simulink model "SimscapeCrane_MPChard"  (R2015b)
settings: Solver=ode15s  StartTime=0.0  StopTime=T  RelTol=1e-3
values from neighbouring files (symbols this model uses):
  m = m1/N    [ConstraintMatrices.m]
  N = N1/(n+c)    [SoftPadding.m]    (also in testMPC.m = ceil(Tf/Ts); testMyLP.m = ceil(1.5/Ts); testRHC.m = ceil(1.5/Ts))
  s = size(A)    [Prediction.m]
  Ts = 1.5/10    (= 0.15)    [testMPC.m]    (also in testMyLP.m; testRHC.m)
  xTarget = [xRange(2)*0.8 0 xRange(2)*0.8 0 0 0 0 0]'    [testMyLP.m]
  xZero = xRange(2)*0.05    [testMPC.m]    (also in testRHC.m = 0)
  yZero = yRange(2)*0.05    [testMPC.m]    (also in testRHC.m = 0)
undefined symbols (not defined in the file or in its folder): Al, blx0, blxe, CD, Dx0, MR, TxBreak, TxCoulomb, TxVisc, TyBreak, TyCoulomb, TzBreak, TzCoulomb, ucon, X, xRange, Y, yRange, Z, zRange, zZero
undefined symbols (not defined in the file): M, TorqueMultX, TorqueMultY, TorqueMultZ, TxTrans, TyTrans, TyVisc, TzTrans, TzVisc
libraries: sm_lib x146, fl_lib x62, nesl_utility x24, elec_lib x9, simulink x6, sm_double_wishbone_suspension_lib x4, aerolibtransform2 x1
(part 14 of 14)

== system SimscapeCrane_MPChard/Crane1/XY actuator/DC Y/PWM & H-Bridge1/Vr Scope ==
  Electrical Reference1 : fl_lib/Electrical/Electrical Elements/Electrical Reference
  PS-Simulink Converter 2 : nesl_utility/PS-Simulink Converter  PhysicalDomain=network_engine_domain  SubClassName=ps_output  LeftPortType=input  RightPortType=output  PseudoPeriodic=off  Frequencies=[]  Unit=V  AffineConversion=off
  Voltage Sensor : fl_lib/Electrical/Electrical Sensors/Voltage Sensor
  Vr : Scope
  u : PMIOPort  Port=1  Side=Left
  wires:
  PS-Simulink Converter 2/1 -> Vr/1
  connections:
  u/RConn1 -- Voltage Sensor/LConn1
  Voltage Sensor/RConn1 -- PS-Simulink Converter 2/LConn1
  Voltage Sensor/RConn2 -- Electrical Reference1/LConn1

== system SimscapeCrane_MPChard/Crane1/XY actuator/X rail/DC X/PWM & H-Bridge ==
  note: For validation purposes the simulation mode
      | can be set to PWM in both the Controlled PWM
      | and H-Bridge blocks.
  Controlled PWM Voltage : elec_lib/Actuators & Drivers/Drivers/Controlled PWM Voltage  F=10000 Hz  TD=0 s  pulse_width_offset=0 s  Vmin=0 V  Vmax=5 V  Vm=5 V  pwm_or_av=2  event_type=1  sample_time=1e-6 s
  Electrical Reference2 : fl_lib/Electrical/Electrical Elements/Electrical Reference
  H-Bridge : elec_lib/Actuators & Drivers/Drivers/H-Bridge  Venable=2.5 V  Vmax=5 V  Vreverse=2.5 V  Vbrake=2.5 V  Vm=24 V  pwm_or_av=2  discontinuous=0  freewheeling_mode=1  freewheeling_mode_disc=1  Ron=0.1 Ohm  Don=0.1 Ohm  Rload=10 Ohm  Lload=1e-5 H  F=10 kHz  thermal_mass=100 J/K  initial_temperature=298.15 K  Ron2=0.1 Ohm  Don2=0.05 Ohm  Tmeas=298.15 K  Tmeas2=398.15 K
  PWM Scope : Subsystem
  REV Scope : Subsystem  Commented=on
  Vr Scope : Subsystem  Commented=on
  V+ : PMIOPort  Port=1  Side=Right
  V- : PMIOPort  Port=2  Side=Right
  Vr : PMIOPort  Port=3  Side=Left
  REV : PMIOPort  Port=4  Side=Left
  "brk " : PMIOPort  Port=5  Side=Left
  "gnd " : PMIOPort  Port=6  Side=Left
  connections:
  V+/RConn1 -- H-Bridge/RConn1
  H-Bridge/RConn2 -- V-/RConn1 -- Electrical Reference2/LConn1
  PWM Scope/LConn1 -- H-Bridge/LConn1 -- Controlled PWM Voltage/RConn1
  Vr Scope/LConn1 -- Controlled PWM Voltage/LConn1 -- Vr/RConn1
  REV Scope/LConn1 -- H-Bridge/LConn3 -- REV/RConn1
  H-Bridge/LConn2 -- Controlled PWM Voltage/RConn2 -- Controlled PWM Voltage/LConn2 -- "gnd "/RConn1
  "brk "/RConn1 -- H-Bridge/LConn4

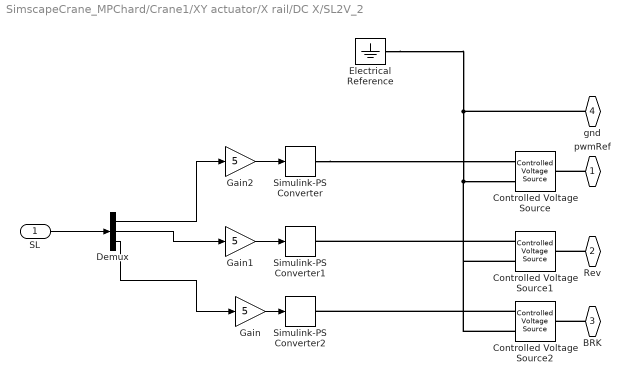
== system SimscapeCrane_MPChard/Crane1/XY actuator/X rail/DC X/SL2V_2 ==
  SL : Inport
  Controlled Voltage Source : fl_lib/Electrical/Electrical Sources/Controlled Voltage Source
  Controlled Voltage Source1 : fl_lib/Electrical/Electrical Sources/Controlled Voltage Source
  Controlled Voltage Source2 : fl_lib/Electrical/Electrical Sources/Controlled Voltage Source
  Demux : Demux  Outputs=3
  Electrical Reference : fl_lib/Electrical/Electrical Elements/Electrical Reference
  Gain : Gain  Gain=5
  Gain1 : Gain  Gain=5
  Gain2 : Gain  Gain=5
  Simulink-PS Converter : nesl_utility/Simulink-PS Converter  PhysicalDomain=network_engine_domain  SubClassName=ps_input  LeftPortType=input  RightPortType=output  PseudoPeriodic=off  Frequencies=[]  NoiseDistribution=none  NoiseParameters=[]  Unit=V  AffineConversion=off  InputFiltering=off  SimscapeFilterOrder=1  InputFilterTimeConstant=.001  UdotUserProvided=0
  Simulink-PS Converter1 : nesl_utility/Simulink-PS Converter  PhysicalDomain=network_engine_domain  SubClassName=ps_input  LeftPortType=input  RightPortType=output  PseudoPeriodic=off  Frequencies=[]  NoiseDistribution=none  NoiseParameters=[]  Unit=V  AffineConversion=off  InputFiltering=off  SimscapeFilterOrder=1  InputFilterTimeConstant=.001  UdotUserProvided=0
  Simulink-PS Converter2 : nesl_utility/Simulink-PS Converter  PhysicalDomain=network_engine_domain  SubClassName=ps_input  LeftPortType=input  RightPortType=output  PseudoPeriodic=off  Frequencies=[]  NoiseDistribution=none  NoiseParameters=[]  Unit=V  AffineConversion=off  InputFiltering=off  SimscapeFilterOrder=1  InputFilterTimeConstant=.001  UdotUserProvided=0
  pwmRef : PMIOPort  Port=1  Side=Right
  Rev : PMIOPort  Port=2  Side=Right
  BRK : PMIOPort  Port=3  Side=Right
  "gnd " : PMIOPort  Port=4  Side=Right
  wires:
  SL/1 -> Demux/1
  Demux/1 -> Gain2/1
  Demux/3 -> Gain/1
  Gain/1 -> Simulink-PS Converter2/1
  Demux/2 -> Gain1/1
  Gain1/1 -> Simulink-PS Converter1/1
  Gain2/1 -> Simulink-PS Converter/1
  connections:
  Simulink-PS Converter/RConn1 -- Controlled Voltage Source/RConn1
  pwmRef/RConn1 -- Controlled Voltage Source/LConn1
  Electrical Reference/LConn1 -- "gnd "/RConn1 -- Controlled Voltage Source/RConn2 -- Controlled Voltage Source1/RConn2 -- Controlled Voltage Source2/RConn2
  Rev/RConn1 -- Controlled Voltage Source1/LConn1
  Controlled Voltage Source2/RConn1 -- Simulink-PS Converter2/RConn1
  BRK/RConn1 -- Controlled Voltage Source2/LConn1
  Controlled Voltage Source1/RConn1 -- Simulink-PS Converter1/RConn1

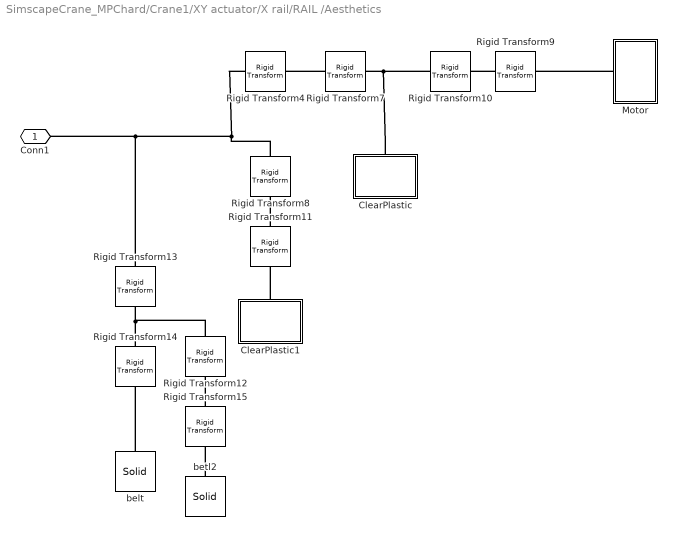
== system SimscapeCrane_MPChard/Crane1/XY actuator/X rail/RAIL /Aesthetics ==
  ClearPlastic : Subsystem
  ClearPlastic1 : Subsystem
  Motor : Subsystem
  Rigid Transform10 : sm_lib/Frames and Transforms/Rigid Transform  TranslationMethod=StandardAxis  TranslationLengthUnit=m  TranslationStandardAxis=+X  TranslationStandardOffset=0.03  TranslationCartesianOffset="[-0.5 0  0]"  TranslationROffset=0  TranslationROffsetUnits=m  TranslationZOffset=0  TranslationZOffsetUnits=m  TranslationThetaOffset=0  TranslationThetaOffsetUnits=deg  RotationMethod=None  RotationAngleUnits=deg  RotationStandardAxis=+Y  RotationAngle=90  RotationArbitraryAxis=[0 0 1]  FollAlignAxisA=+X  BaseAlignAxisA=+Y  FollAlignAxisB=+Y  BaseAlignAxisB=+Z  RotationSequenceAxes=FollowerAxes  RotationSequence=XYX  RotationSequenceAngles=[0 0 0]  RotationSequenceAnglesUnits=deg  RotationMatrix=[1 0 0; 0 1 0; 0 0 1]  BlockFunction=simmechanics.library.frames_transforms.rigid_transform
  Rigid Transform11 : sm_lib/Frames and Transforms/Rigid Transform  TranslationMethod=StandardAxis  TranslationLengthUnit=m  TranslationStandardAxis=-Z  TranslationStandardOffset=0.05  TranslationCartesianOffset="[-0.5 0  0]"  TranslationROffset=0  TranslationROffsetUnits=m  TranslationZOffset=0  TranslationZOffsetUnits=m  TranslationThetaOffset=0  TranslationThetaOffsetUnits=deg  RotationMethod=None  RotationAngleUnits=deg  RotationStandardAxis=+Y  RotationAngle=90  RotationArbitraryAxis=[0 0 1]  FollAlignAxisA=+X  BaseAlignAxisA=+Y  FollAlignAxisB=+Y  BaseAlignAxisB=+Z  RotationSequenceAxes=FollowerAxes  RotationSequence=XYX  RotationSequenceAngles=[0 0 0]  RotationSequenceAnglesUnits=deg  RotationMatrix=[1 0 0; 0 1 0; 0 0 1]  BlockFunction=simmechanics.library.frames_transforms.rigid_transform
  Rigid Transform12 : sm_lib/Frames and Transforms/Rigid Transform  TranslationMethod=StandardAxis  TranslationLengthUnit=m  TranslationStandardAxis=-Z  TranslationStandardOffset=0.06  TranslationCartesianOffset="[-0.5 0  0]"  TranslationROffset=0  TranslationROffsetUnits=m  TranslationZOffset=0  TranslationZOffsetUnits=m  TranslationThetaOffset=0  TranslationThetaOffsetUnits=deg  RotationMethod=None  RotationAngleUnits=deg  RotationStandardAxis=+Y  RotationAngle=90  RotationArbitraryAxis=[0 0 1]  FollAlignAxisA=+X  BaseAlignAxisA=+Y  FollAlignAxisB=+Y  BaseAlignAxisB=+Z  RotationSequenceAxes=FollowerAxes  RotationSequence=XYX  RotationSequenceAngles=[0 0 0]  RotationSequenceAnglesUnits=deg  RotationMatrix=[1 0 0; 0 1 0; 0 0 1]  BlockFunction=simmechanics.library.frames_transforms.rigid_transform
  Rigid Transform13 : sm_lib/Frames and Transforms/Rigid Transform  TranslationMethod=StandardAxis  TranslationLengthUnit=m  TranslationStandardAxis=-X  TranslationStandardOffset=0.04  TranslationCartesianOffset="[-0.5 0  0]"  TranslationROffset=0  TranslationROffsetUnits=m  TranslationZOffset=0  TranslationZOffsetUnits=m  TranslationThetaOffset=0  TranslationThetaOffsetUnits=deg  RotationMethod=None  RotationAngleUnits=deg  RotationStandardAxis=+Y  RotationAngle=90  RotationArbitraryAxis=[0 0 1]  FollAlignAxisA=+X  BaseAlignAxisA=+Y  FollAlignAxisB=+Y  BaseAlignAxisB=+Z  RotationSequenceAxes=FollowerAxes  RotationSequence=XYX  RotationSequenceAngles=[0 0 0]  RotationSequenceAnglesUnits=deg  RotationMatrix=[1 0 0; 0 1 0; 0 0 1]  BlockFunction=simmechanics.library.frames_transforms.rigid_transform
  Rigid Transform14 : sm_lib/Frames and Transforms/Rigid Transform  TranslationMethod=None  TranslationLengthUnit=m  TranslationStandardAxis=-Z  TranslationStandardOffset=0.04  TranslationCartesianOffset="[-0.5 0  0]"  TranslationROffset=0  TranslationROffsetUnits=m  TranslationZOffset=0  TranslationZOffsetUnits=m  TranslationThetaOffset=0  TranslationThetaOffsetUnits=deg  RotationMethod=StandardAxis  RotationAngleUnits=deg  RotationStandardAxis=+Z  RotationAngle=90  RotationArbitraryAxis=[0 0 1]  FollAlignAxisA=+X  BaseAlignAxisA=+Y  FollAlignAxisB=+Y  BaseAlignAxisB=+Z  RotationSequenceAxes=FollowerAxes  RotationSequence=XYX  RotationSequenceAngles=[0 0 0]  RotationSequenceAnglesUnits=deg  RotationMatrix=[1 0 0; 0 1 0; 0 0 1]  BlockFunction=simmechanics.library.frames_transforms.rigid_transform
  Rigid Transform15 : sm_lib/Frames and Transforms/Rigid Transform  TranslationMethod=None  TranslationLengthUnit=m  TranslationStandardAxis=-Z  TranslationStandardOffset=0.04  TranslationCartesianOffset="[-0.5 0  0]"  TranslationROffset=0  TranslationROffsetUnits=m  TranslationZOffset=0  TranslationZOffsetUnits=m  TranslationThetaOffset=0  TranslationThetaOffsetUnits=deg  RotationMethod=StandardAxis  RotationAngleUnits=deg  RotationStandardAxis=+Z  RotationAngle=90  RotationArbitraryAxis=[0 0 1]  FollAlignAxisA=+X  BaseAlignAxisA=+Y  FollAlignAxisB=+Y  BaseAlignAxisB=+Z  RotationSequenceAxes=FollowerAxes  RotationSequence=XYX  RotationSequenceAngles=[0 0 0]  RotationSequenceAnglesUnits=deg  RotationMatrix=[1 0 0; 0 1 0; 0 0 1]  BlockFunction=simmechanics.library.frames_transforms.rigid_transform
  Rigid Transform4 : sm_lib/Frames and Transforms/Rigid Transform  TranslationMethod=StandardAxis  TranslationLengthUnit=m  TranslationStandardAxis=-Y  TranslationStandardOffset=0.56  TranslationCartesianOffset="[-0.5 0  0]"  TranslationROffset=0  TranslationROffsetUnits=m  TranslationZOffset=0  TranslationZOffsetUnits=m  TranslationThetaOffset=0  TranslationThetaOffsetUnits=deg  RotationMethod=None  RotationAngleUnits=deg  RotationStandardAxis=+Y  RotationAngle=90  RotationArbitraryAxis=[0 0 1]  FollAlignAxisA=+X  BaseAlignAxisA=+Y  FollAlignAxisB=+Y  BaseAlignAxisB=+Z  RotationSequenceAxes=FollowerAxes  RotationSequence=XYX  RotationSequenceAngles=[0 0 0]  RotationSequenceAnglesUnits=deg  RotationMatrix=[1 0 0; 0 1 0; 0 0 1]  BlockFunction=simmechanics.library.frames_transforms.rigid_transform
  Rigid Transform7 : sm_lib/Frames and Transforms/Rigid Transform  TranslationMethod=StandardAxis  TranslationLengthUnit=m  TranslationStandardAxis=-Z  TranslationStandardOffset=0.05  TranslationCartesianOffset="[-0.5 0  0]"  TranslationROffset=0  TranslationROffsetUnits=m  TranslationZOffset=0  TranslationZOffsetUnits=m  TranslationThetaOffset=0  TranslationThetaOffsetUnits=deg  RotationMethod=None  RotationAngleUnits=deg  RotationStandardAxis=+Y  RotationAngle=90  RotationArbitraryAxis=[0 0 1]  FollAlignAxisA=+X  BaseAlignAxisA=+Y  FollAlignAxisB=+Y  BaseAlignAxisB=+Z  RotationSequenceAxes=FollowerAxes  RotationSequence=XYX  RotationSequenceAngles=[0 0 0]  RotationSequenceAnglesUnits=deg  RotationMatrix=[1 0 0; 0 1 0; 0 0 1]  BlockFunction=simmechanics.library.frames_transforms.rigid_transform
  Rigid Transform8 : sm_lib/Frames and Transforms/Rigid Transform  TranslationMethod=StandardAxis  TranslationLengthUnit=m  TranslationStandardAxis=+Y  TranslationStandardOffset=0.56  TranslationCartesianOffset="[-0.5 0  0]"  TranslationROffset=0  TranslationROffsetUnits=m  TranslationZOffset=0  TranslationZOffsetUnits=m  TranslationThetaOffset=0  TranslationThetaOffsetUnits=deg  RotationMethod=None  RotationAngleUnits=deg  RotationStandardAxis=+Y  RotationAngle=90  RotationArbitraryAxis=[0 0 1]  FollAlignAxisA=+X  BaseAlignAxisA=+Y  FollAlignAxisB=+Y  BaseAlignAxisB=+Z  RotationSequenceAxes=FollowerAxes  RotationSequence=XYX  RotationSequenceAngles=[0 0 0]  RotationSequenceAnglesUnits=deg  RotationMatrix=[1 0 0; 0 1 0; 0 0 1]  BlockFunction=simmechanics.library.frames_transforms.rigid_transform
  Rigid Transform9 : sm_lib/Frames and Transforms/Rigid Transform  TranslationMethod=None  TranslationLengthUnit=m  TranslationStandardAxis=-Z  TranslationStandardOffset=0.05  TranslationCartesianOffset="[-0.5 0  0]"  TranslationROffset=0  TranslationROffsetUnits=m  TranslationZOffset=0  TranslationZOffsetUnits=m  TranslationThetaOffset=0  TranslationThetaOffsetUnits=deg  RotationMethod=StandardAxis  RotationAngleUnits=deg  RotationStandardAxis=+Z  RotationAngle=90  RotationArbitraryAxis=[0 0 1]  FollAlignAxisA=+X  BaseAlignAxisA=+Y  FollAlignAxisB=+Y  BaseAlignAxisB=+Z  RotationSequenceAxes=FollowerAxes  RotationSequence=XYX  RotationSequenceAngles=[0 0 0]  RotationSequenceAnglesUnits=deg  RotationMatrix=[1 0 0; 0 1 0; 0 0 1]  BlockFunction=simmechanics.library.frames_transforms.rigid_transform
  belt : sm_lib/Body Elements/Solid  InertiaType=PointMass  Mass=0  MassUnits=kg  CenterOfMass=[0 0 0]  CenterOfMassUnits=m  MomentsOfInertia=[1 1 1]  MomentsOfInertiaUnits=kg*m^2  ProductsOfInertia=[0 0 0]  ProductsOfInertiaUnits=kg*m^2  DensityBased=off  Density=1000  DensityUnits=kg/(m^3)  DoExposeReferenceFrame=on  SerializedFrames=<Frames/>  GraphicType=FromGeometry  MarkerShape=Sphere  MarkerSize=10  MarkerSizeUnits=m  GraphicVisPropType=SimpleVisualProperties  GraphicDiffuseColor=[0.0 0.0 0.8]  GraphicSpecularColor=[0.5 0.5 0.5 1.0]  GraphicAmbientColor=[0.15 0.15 0.15 1.0]  GraphicEmissiveColor=[0.0 0.0 0.0 1.0]  GraphicShininess=100  GraphicOpacity=1.0  GeometryShape=Brick  RectangleSize=[1 1]  RectangleSizeUnits=m  BrickDimensions=[1.2 0.001 0.001]  BrickDimensionUnits=m  CylinderRadius=0.02  CylinderRadiusUnits=m  CylinderLength=1  CylinderLengthUnits=m  SphereRadius=1  SphereRadiusUnits=m  EllipsoidRadii=[1 1 1]  EllipsoidRadiiUnits=m  ExtrusionCrossSection=[1 1; -1 1; -1 -1; 1 -1]  ExtrusionCrossSectionUnits=m  ExtrusionLength=1  ExtrusionLengthUnits=m  PolygonNumSides=3  PolygonOuterRadius=1  PolygonOuterRadiusUnits=m  ExtGeomFileType=STL  ExtGeomFileUnits=m  RevolutionCrossSection=[1 1; 1 -1; 2 -1; 2 1]  RevolutionCrossSectionUnits=m  RevolutionExtent=Full  RevolutionAngle=180  RevolutionAngleUnits=deg  BlockFunction=simmechanics.library.body_elements.solid
  "betl2 " : sm_lib/Body Elements/Solid  InertiaType=PointMass  Mass=0  MassUnits=kg  CenterOfMass=[0 0 0]  CenterOfMassUnits=m  MomentsOfInertia=[1 1 1]  MomentsOfInertiaUnits=kg*m^2  ProductsOfInertia=[0 0 0]  ProductsOfInertiaUnits=kg*m^2  DensityBased=off  Density=1000  DensityUnits=kg/(m^3)  DoExposeReferenceFrame=on  SerializedFrames=<Frames/>  GraphicType=FromGeometry  MarkerShape=Sphere  MarkerSize=10  MarkerSizeUnits=m  GraphicVisPropType=SimpleVisualProperties  GraphicDiffuseColor=[0.0 0.0 0.8]  GraphicSpecularColor=[0.5 0.5 0.5 1.0]  GraphicAmbientColor=[0.15 0.15 0.15 1.0]  GraphicEmissiveColor=[0.0 0.0 0.0 1.0]  GraphicShininess=100  GraphicOpacity=1.0  GeometryShape=Brick  RectangleSize=[1 1]  RectangleSizeUnits=m  BrickDimensions=[1.2 0.001 0.001]  BrickDimensionUnits=m  CylinderRadius=0.02  CylinderRadiusUnits=m  CylinderLength=1  CylinderLengthUnits=m  SphereRadius=1  SphereRadiusUnits=m  EllipsoidRadii=[1 1 1]  EllipsoidRadiiUnits=m  ExtrusionCrossSection=[1 1; -1 1; -1 -1; 1 -1]  ExtrusionCrossSectionUnits=m  ExtrusionLength=1  ExtrusionLengthUnits=m  PolygonNumSides=3  PolygonOuterRadius=1  PolygonOuterRadiusUnits=m  ExtGeomFileType=STL  ExtGeomFileUnits=m  RevolutionCrossSection=[1 1; 1 -1; 2 -1; 2 1]  RevolutionCrossSectionUnits=m  RevolutionExtent=Full  RevolutionAngle=180  RevolutionAngleUnits=deg  BlockFunction=simmechanics.library.body_elements.solid
  Conn1 : PMIOPort  Port=1  Side=Left
  connections:
  Rigid Transform10/LConn1 -- ClearPlastic/RConn1 -- Rigid Transform7/RConn1
  Rigid Transform13/RConn1 -- Rigid Transform14/LConn1 -- Rigid Transform12/LConn1
  Motor/LConn1 -- Rigid Transform9/RConn1
  Rigid Transform7/LConn1 -- Rigid Transform4/RConn1
  ClearPlastic1/RConn1 -- Rigid Transform11/RConn1
  Rigid Transform11/LConn1 -- Rigid Transform8/RConn1
  Rigid Transform15/LConn1 -- Rigid Transform12/RConn1
  "betl2 "/RConn1 -- Rigid Transform15/RConn1
  Rigid Transform8/LConn1 -- Rigid Transform13/LConn1 -- Conn1/RConn1 -- Rigid Transform4/LConn1
  belt/RConn1 -- Rigid Transform14/RConn1
  Rigid Transform9/LConn1 -- Rigid Transform10/RConn1

== system SimscapeCrane_MPChard/Crane1/XY actuator/Y cart/CART/Motor ==
  Cart2 : sm_lib/Body Elements/Solid  InertiaType=PointMass  Mass=0  MassUnits=kg  CenterOfMass=[0 0 0]  CenterOfMassUnits=m  MomentsOfInertia=[1 1 1]  MomentsOfInertiaUnits=kg*m^2  ProductsOfInertia=[0 0 0]  ProductsOfInertiaUnits=kg*m^2  DensityBased=off  Density=1000  DensityUnits=kg/(m^3)  DoExposeReferenceFrame=on  SerializedFrames=<Frames/>  GraphicType=FromGeometry  MarkerShape=Sphere  MarkerSize=10  MarkerSizeUnits=m  GraphicVisPropType=AdvancedVisualProperties  GraphicDiffuseColor=[0.1 0.1 0.0]  GraphicSpecularColor=[0.5 0.5 0.5 1.0]  GraphicAmbientColor=[0.15 0.2 0.3 1.0]  GraphicEmissiveColor=[0.0 0.0 0.0 1.0]  GraphicShininess=30  GraphicOpacity=1.0  GeometryShape=Cylinder  RectangleSize=[1 1]  RectangleSizeUnits=m  BrickDimensions=[0.06 0.12 0.12]  BrickDimensionUnits=m  CylinderRadius=1.7  CylinderRadiusUnits=cm  CylinderLength=6  CylinderLengthUnits=cm  SphereRadius=1  SphereRadiusUnits=m  EllipsoidRadii=[1 1 1]  EllipsoidRadiiUnits=m  ExtrusionCrossSection=[1 1; -1 1; -1 -1; 1 -1]  ExtrusionCrossSectionUnits=m  ExtrusionLength=1  ExtrusionLengthUnits=m  PolygonNumSides=3  PolygonOuterRadius=1  PolygonOuterRadiusUnits=m  ExtGeomFileType=STL  ExtGeomFileUnits=m  RevolutionCrossSection=[1 1; 1 -1; 2 -1; 2 1]  RevolutionCrossSectionUnits=m  RevolutionExtent=Full  RevolutionAngle=180  RevolutionAngleUnits=deg  BlockFunction=simmechanics.library.body_elements.solid
  Cart3 : sm_lib/Body Elements/Solid  InertiaType=PointMass  Mass=0  MassUnits=kg  CenterOfMass=[0 0 0]  CenterOfMassUnits=m  MomentsOfInertia=[1 1 1]  MomentsOfInertiaUnits=kg*m^2  ProductsOfInertia=[0 0 0]  ProductsOfInertiaUnits=kg*m^2  DensityBased=off  Density=1000  DensityUnits=kg/(m^3)  DoExposeReferenceFrame=on  SerializedFrames=<Frames/>  GraphicType=FromGeometry  MarkerShape=Sphere  MarkerSize=10  MarkerSizeUnits=m  GraphicVisPropType=SimpleVisualProperties  GraphicDiffuseColor=[0.4 0.4 0.4]  GraphicSpecularColor=[0.5 0.5 0.5 1.0]  GraphicAmbientColor=[0.15 0.15 0.15 1.0]  GraphicEmissiveColor=[0.0 0.0 0.0 1.0]  GraphicShininess=75  GraphicOpacity=1.0  GeometryShape=Cylinder  RectangleSize=[1 1]  RectangleSizeUnits=m  BrickDimensions=[0.06 0.12 0.12]  BrickDimensionUnits=m  CylinderRadius=2.6  CylinderRadiusUnits=cm  CylinderLength=3  CylinderLengthUnits=cm  SphereRadius=1  SphereRadiusUnits=m  EllipsoidRadii=[1 1 1]  EllipsoidRadiiUnits=m  ExtrusionCrossSection=[1 1; -1 1; -1 -1; 1 -1]  ExtrusionCrossSectionUnits=m  ExtrusionLength=1  ExtrusionLengthUnits=m  PolygonNumSides=3  PolygonOuterRadius=1  PolygonOuterRadiusUnits=m  ExtGeomFileType=STL  ExtGeomFileUnits=m  RevolutionCrossSection=[1 1; 1 -1; 2 -1; 2 1]  RevolutionCrossSectionUnits=m  RevolutionExtent=Full  RevolutionAngle=180  RevolutionAngleUnits=deg  BlockFunction=simmechanics.library.body_elements.solid
  Rigid Transform3 : sm_lib/Frames and Transforms/Rigid Transform  TranslationMethod=None  TranslationLengthUnit=m  TranslationStandardAxis=-X  TranslationStandardOffset=0.04  TranslationCartesianOffset="[-0.5 0  0]"  TranslationROffset=0  TranslationROffsetUnits=m  TranslationZOffset=0  TranslationZOffsetUnits=m  TranslationThetaOffset=0  TranslationThetaOffsetUnits=deg  RotationMethod=StandardAxis  RotationAngleUnits=deg  RotationStandardAxis=-X  RotationAngle=90  RotationArbitraryAxis=[0 0 1]  FollAlignAxisA=+X  BaseAlignAxisA=+Y  FollAlignAxisB=+Y  BaseAlignAxisB=+Z  RotationSequenceAxes=FollowerAxes  RotationSequence=XYX  RotationSequenceAngles=[0 0 0]  RotationSequenceAnglesUnits=deg  RotationMatrix=[1 0 0; 0 1 0; 0 0 1]  BlockFunction=simmechanics.library.frames_transforms.rigid_transform
  Rigid Transform4 : sm_lib/Frames and Transforms/Rigid Transform  TranslationMethod=None  TranslationLengthUnit=m  TranslationStandardAxis=-X  TranslationStandardOffset=0.04  TranslationCartesianOffset="[-0.5 0  0]"  TranslationROffset=0  TranslationROffsetUnits=m  TranslationZOffset=0  TranslationZOffsetUnits=m  TranslationThetaOffset=0  TranslationThetaOffsetUnits=deg  RotationMethod=StandardAxis  RotationAngleUnits=deg  RotationStandardAxis=-X  RotationAngle=90  RotationArbitraryAxis=[0 0 1]  FollAlignAxisA=+X  BaseAlignAxisA=+Y  FollAlignAxisB=+Y  BaseAlignAxisB=+Z  RotationSequenceAxes=FollowerAxes  RotationSequence=XYX  RotationSequenceAngles=[0 0 0]  RotationSequenceAnglesUnits=deg  RotationMatrix=[1 0 0; 0 1 0; 0 0 1]  BlockFunction=simmechanics.library.frames_transforms.rigid_transform
  Rigid Transform5 : sm_lib/Frames and Transforms/Rigid Transform  TranslationMethod=StandardAxis  TranslationLengthUnit=m  TranslationStandardAxis=-Y  TranslationStandardOffset=0.015  TranslationCartesianOffset="[-0.5 0  0]"  TranslationROffset=0  TranslationROffsetUnits=m  TranslationZOffset=0  TranslationZOffsetUnits=m  TranslationThetaOffset=0  TranslationThetaOffsetUnits=deg  RotationMethod=None  RotationAngleUnits=deg  RotationStandardAxis=-X  RotationAngle=90  RotationArbitraryAxis=[0 0 1]  FollAlignAxisA=+X  BaseAlignAxisA=+Y  FollAlignAxisB=+Y  BaseAlignAxisB=+Z  RotationSequenceAxes=FollowerAxes  RotationSequence=XYX  RotationSequenceAngles=[0 0 0]  RotationSequenceAnglesUnits=deg  RotationMatrix=[1 0 0; 0 1 0; 0 0 1]  BlockFunction=simmechanics.library.frames_transforms.rigid_transform
  Rigid Transform6 : sm_lib/Frames and Transforms/Rigid Transform  TranslationMethod=StandardAxis  TranslationLengthUnit=m  TranslationStandardAxis=+Y  TranslationStandardOffset=0.03  TranslationCartesianOffset="[-0.5 0  0]"  TranslationROffset=0  TranslationROffsetUnits=m  TranslationZOffset=0  TranslationZOffsetUnits=m  TranslationThetaOffset=0  TranslationThetaOffsetUnits=deg  RotationMethod=None  RotationAngleUnits=deg  RotationStandardAxis=-X  RotationAngle=90  RotationArbitraryAxis=[0 0 1]  FollAlignAxisA=+X  BaseAlignAxisA=+Y  FollAlignAxisB=+Y  BaseAlignAxisB=+Z  RotationSequenceAxes=FollowerAxes  RotationSequence=XYX  RotationSequenceAngles=[0 0 0]  RotationSequenceAnglesUnits=deg  RotationMatrix=[1 0 0; 0 1 0; 0 0 1]  BlockFunction=simmechanics.library.frames_transforms.rigid_transform
  Conn1 : PMIOPort  Port=1  Side=Left
  connections:
  Rigid Transform3/RConn1 -- Cart2/RConn1
  Rigid Transform4/RConn1 -- Cart3/RConn1
  Rigid Transform6/LConn1 -- Conn1/RConn1 -- Rigid Transform5/LConn1
  Rigid Transform6/RConn1 -- Rigid Transform4/LConn1
  Rigid Transform5/RConn1 -- Rigid Transform3/LConn1

== system SimscapeCrane_MPChard/Crane1/XY actuator/X rail/DC X/PWM & H-Bridge/PWM Scope ==
  Electrical Reference1 : fl_lib/Electrical/Electrical Elements/Electrical Reference
  PS-Simulink Converter 2 : nesl_utility/PS-Simulink Converter  PhysicalDomain=network_engine_domain  SubClassName=ps_output  LeftPortType=input  RightPortType=output  PseudoPeriodic=off  Frequencies=[]  Unit=V  AffineConversion=off
  PWM : Scope
  Voltage Sensor : fl_lib/Electrical/Electrical Sensors/Voltage Sensor
  u : PMIOPort  Port=1  Side=Left
  wires:
  PS-Simulink Converter 2/1 -> PWM/1
  connections:
  Voltage Sensor/RConn2 -- Electrical Reference1/LConn1
  Voltage Sensor/RConn1 -- PS-Simulink Converter 2/LConn1
  u/RConn1 -- Voltage Sensor/LConn1

== system SimscapeCrane_MPChard/Crane1/XY actuator/X rail/DC X/PWM & H-Bridge/REV Scope ==
  Electrical Reference1 : fl_lib/Electrical/Electrical Elements/Electrical Reference
  PS-Simulink Converter 2 : nesl_utility/PS-Simulink Converter  PhysicalDomain=network_engine_domain  SubClassName=ps_output  LeftPortType=input  RightPortType=output  PseudoPeriodic=off  Frequencies=[]  Unit=V  AffineConversion=off
  REV : Scope
  Voltage Sensor : fl_lib/Electrical/Electrical Sensors/Voltage Sensor
  u : PMIOPort  Port=1  Side=Left
  wires:
  PS-Simulink Converter 2/1 -> REV/1
  connections:
  Voltage Sensor/RConn2 -- Electrical Reference1/LConn1
  Voltage Sensor/RConn1 -- PS-Simulink Converter 2/LConn1
  u/RConn1 -- Voltage Sensor/LConn1

== system SimscapeCrane_MPChard/Crane1/XY actuator/X rail/DC X/PWM & H-Bridge/Vr Scope ==
  Electrical Reference1 : fl_lib/Electrical/Electrical Elements/Electrical Reference
  PS-Simulink Converter 2 : nesl_utility/PS-Simulink Converter  PhysicalDomain=network_engine_domain  SubClassName=ps_output  LeftPortType=input  RightPortType=output  PseudoPeriodic=off  Frequencies=[]  Unit=V  AffineConversion=off
  Voltage Sensor : fl_lib/Electrical/Electrical Sensors/Voltage Sensor
  Vr : Scope
  u : PMIOPort  Port=1  Side=Left
  wires:
  PS-Simulink Converter 2/1 -> Vr/1
  connections:
  u/RConn1 -- Voltage Sensor/LConn1
  Voltage Sensor/RConn1 -- PS-Simulink Converter 2/LConn1
  Voltage Sensor/RConn2 -- Electrical Reference1/LConn1

== system SimscapeCrane_MPChard/Crane1/XY actuator/X rail/RAIL /Aesthetics/ClearPlastic ==
  Rail2 : sm_lib/Body Elements/Solid  InertiaType=PointMass  Mass=0  MassUnits=kg  CenterOfMass=[0 0 0]  CenterOfMassUnits=m  MomentsOfInertia=[1 1 1]  MomentsOfInertiaUnits=kg*m^2  ProductsOfInertia=[0 0 0]  ProductsOfInertiaUnits=kg*m^2  DensityBased=off  Density=1000  DensityUnits=kg/(m^3)  DoExposeReferenceFrame=on  SerializedFrames=<Frames/>  GraphicType=FromGeometry  MarkerShape=Sphere  MarkerSize=10  MarkerSizeUnits=m  GraphicVisPropType=SimpleVisualProperties  GraphicDiffuseColor=[0.8 0.8 0.8]  GraphicSpecularColor=[0.5 0.5 0.5 1.0]  GraphicAmbientColor=[0.15 0.15 0.15 1.0]  GraphicEmissiveColor=[0.0 0.0 0.0 1.0]  GraphicShininess=100  GraphicOpacity=0.4  GeometryShape=Brick  RectangleSize=[1 1]  RectangleSizeUnits=m  BrickDimensions=[0.05 0.09 0.015]  BrickDimensionUnits=m  CylinderRadius=0.02  CylinderRadiusUnits=m  CylinderLength=1  CylinderLengthUnits=m  SphereRadius=1  SphereRadiusUnits=m  EllipsoidRadii=[1 1 1]  EllipsoidRadiiUnits=m  ExtrusionCrossSection=[1 1; -1 1; -1 -1; 1 -1]  ExtrusionCrossSectionUnits=m  ExtrusionLength=1  ExtrusionLengthUnits=m  PolygonNumSides=3  PolygonOuterRadius=1  PolygonOuterRadiusUnits=m  ExtGeomFileType=STL  ExtGeomFileUnits=m  RevolutionCrossSection=[1 1; 1 -1; 2 -1; 2 1]  RevolutionCrossSectionUnits=m  RevolutionExtent=Full  RevolutionAngle=180  RevolutionAngleUnits=deg  BlockFunction=simmechanics.library.body_elements.solid
  Rigid Transform11 : sm_lib/Frames and Transforms/Rigid Transform  TranslationMethod=None  TranslationLengthUnit=m  TranslationStandardAxis=-Z  TranslationStandardOffset=0.05  TranslationCartesianOffset="[-0.5 0  0]"  TranslationROffset=0  TranslationROffsetUnits=m  TranslationZOffset=0  TranslationZOffsetUnits=m  TranslationThetaOffset=0  TranslationThetaOffsetUnits=deg  RotationMethod=StandardAxis  RotationAngleUnits=deg  RotationStandardAxis=+Z  RotationAngle=90  RotationArbitraryAxis=[0 0 1]  FollAlignAxisA=+X  BaseAlignAxisA=+Y  FollAlignAxisB=+Y  BaseAlignAxisB=+Z  RotationSequenceAxes=FollowerAxes  RotationSequence=XYX  RotationSequenceAngles=[0 0 0]  RotationSequenceAnglesUnits=deg  RotationMatrix=[1 0 0; 0 1 0; 0 0 1]  BlockFunction=simmechanics.library.frames_transforms.rigid_transform
  Rigid Transform12 : sm_lib/Frames and Transforms/Rigid Transform  TranslationMethod=StandardAxis  TranslationLengthUnit=m  TranslationStandardAxis=-X  TranslationStandardOffset=0.03  TranslationCartesianOffset="[-0.5 0  0]"  TranslationROffset=0  TranslationROffsetUnits=m  TranslationZOffset=0  TranslationZOffsetUnits=m  TranslationThetaOffset=0  TranslationThetaOffsetUnits=deg  RotationMethod=None  RotationAngleUnits=deg  RotationStandardAxis=+Y  RotationAngle=90  RotationArbitraryAxis=[0 0 1]  FollAlignAxisA=+X  BaseAlignAxisA=+Y  FollAlignAxisB=+Y  BaseAlignAxisB=+Z  RotationSequenceAxes=FollowerAxes  RotationSequence=XYX  RotationSequenceAngles=[0 0 0]  RotationSequenceAnglesUnits=deg  RotationMatrix=[1 0 0; 0 1 0; 0 0 1]  BlockFunction=simmechanics.library.frames_transforms.rigid_transform
  Rigid Transform8 : sm_lib/Frames and Transforms/Rigid Transform  TranslationMethod=None  TranslationLengthUnit=m  TranslationStandardAxis=-Z  TranslationStandardOffset=0.05  TranslationCartesianOffset="[-0.5 0  0]"  TranslationROffset=0  TranslationROffsetUnits=m  TranslationZOffset=0  TranslationZOffsetUnits=m  TranslationThetaOffset=0  TranslationThetaOffsetUnits=deg  RotationMethod=StandardAxis  RotationAngleUnits=deg  RotationStandardAxis=+X  RotationAngle=90  RotationArbitraryAxis=[0 0 1]  FollAlignAxisA=+X  BaseAlignAxisA=+Y  FollAlignAxisB=+Y  BaseAlignAxisB=+Z  RotationSequenceAxes=FollowerAxes  RotationSequence=XYX  RotationSequenceAngles=[0 0 0]  RotationSequenceAnglesUnits=deg  RotationMatrix=[1 0 0; 0 1 0; 0 0 1]  BlockFunction=simmechanics.library.frames_transforms.rigid_transform
  Conn1 : PMIOPort  Port=1  Side=Right
  connections:
  Rigid Transform12/LConn1 -- Conn1/RConn1
  Rigid Transform8/LConn1 -- Rigid Transform11/RConn1
  Rigid Transform11/LConn1 -- Rigid Transform12/RConn1
  Rigid Transform8/RConn1 -- Rail2/RConn1

== system SimscapeCrane_MPChard/Crane1/XY actuator/X rail/RAIL /Aesthetics/ClearPlastic1 ==
  Rail2 : sm_lib/Body Elements/Solid  InertiaType=PointMass  Mass=0  MassUnits=kg  CenterOfMass=[0 0 0]  CenterOfMassUnits=m  MomentsOfInertia=[1 1 1]  MomentsOfInertiaUnits=kg*m^2  ProductsOfInertia=[0 0 0]  ProductsOfInertiaUnits=kg*m^2  DensityBased=off  Density=1000  DensityUnits=kg/(m^3)  DoExposeReferenceFrame=on  SerializedFrames=<Frames/>  GraphicType=FromGeometry  MarkerShape=Sphere  MarkerSize=10  MarkerSizeUnits=m  GraphicVisPropType=SimpleVisualProperties  GraphicDiffuseColor=[0.8 0.8 0.8]  GraphicSpecularColor=[0.5 0.5 0.5 1.0]  GraphicAmbientColor=[0.15 0.15 0.15 1.0]  GraphicEmissiveColor=[0.0 0.0 0.0 1.0]  GraphicShininess=100  GraphicOpacity=0.4  GeometryShape=Brick  RectangleSize=[1 1]  RectangleSizeUnits=m  BrickDimensions=[0.05 0.09 0.015]  BrickDimensionUnits=m  CylinderRadius=0.02  CylinderRadiusUnits=m  CylinderLength=1  CylinderLengthUnits=m  SphereRadius=1  SphereRadiusUnits=m  EllipsoidRadii=[1 1 1]  EllipsoidRadiiUnits=m  ExtrusionCrossSection=[1 1; -1 1; -1 -1; 1 -1]  ExtrusionCrossSectionUnits=m  ExtrusionLength=1  ExtrusionLengthUnits=m  PolygonNumSides=3  PolygonOuterRadius=1  PolygonOuterRadiusUnits=m  ExtGeomFileType=STL  ExtGeomFileUnits=m  RevolutionCrossSection=[1 1; 1 -1; 2 -1; 2 1]  RevolutionCrossSectionUnits=m  RevolutionExtent=Full  RevolutionAngle=180  RevolutionAngleUnits=deg  BlockFunction=simmechanics.library.body_elements.solid
  Rigid Transform11 : sm_lib/Frames and Transforms/Rigid Transform  TranslationMethod=None  TranslationLengthUnit=m  TranslationStandardAxis=-Z  TranslationStandardOffset=0.05  TranslationCartesianOffset="[-0.5 0  0]"  TranslationROffset=0  TranslationROffsetUnits=m  TranslationZOffset=0  TranslationZOffsetUnits=m  TranslationThetaOffset=0  TranslationThetaOffsetUnits=deg  RotationMethod=StandardAxis  RotationAngleUnits=deg  RotationStandardAxis=+Z  RotationAngle=90  RotationArbitraryAxis=[0 0 1]  FollAlignAxisA=+X  BaseAlignAxisA=+Y  FollAlignAxisB=+Y  BaseAlignAxisB=+Z  RotationSequenceAxes=FollowerAxes  RotationSequence=XYX  RotationSequenceAngles=[0 0 0]  RotationSequenceAnglesUnits=deg  RotationMatrix=[1 0 0; 0 1 0; 0 0 1]  BlockFunction=simmechanics.library.frames_transforms.rigid_transform
  Rigid Transform12 : sm_lib/Frames and Transforms/Rigid Transform  TranslationMethod=StandardAxis  TranslationLengthUnit=m  TranslationStandardAxis=-X  TranslationStandardOffset=0.03  TranslationCartesianOffset="[-0.5 0  0]"  TranslationROffset=0  TranslationROffsetUnits=m  TranslationZOffset=0  TranslationZOffsetUnits=m  TranslationThetaOffset=0  TranslationThetaOffsetUnits=deg  RotationMethod=None  RotationAngleUnits=deg  RotationStandardAxis=+Y  RotationAngle=90  RotationArbitraryAxis=[0 0 1]  FollAlignAxisA=+X  BaseAlignAxisA=+Y  FollAlignAxisB=+Y  BaseAlignAxisB=+Z  RotationSequenceAxes=FollowerAxes  RotationSequence=XYX  RotationSequenceAngles=[0 0 0]  RotationSequenceAnglesUnits=deg  RotationMatrix=[1 0 0; 0 1 0; 0 0 1]  BlockFunction=simmechanics.library.frames_transforms.rigid_transform
  Rigid Transform8 : sm_lib/Frames and Transforms/Rigid Transform  TranslationMethod=None  TranslationLengthUnit=m  TranslationStandardAxis=-Z  TranslationStandardOffset=0.05  TranslationCartesianOffset="[-0.5 0  0]"  TranslationROffset=0  TranslationROffsetUnits=m  TranslationZOffset=0  TranslationZOffsetUnits=m  TranslationThetaOffset=0  TranslationThetaOffsetUnits=deg  RotationMethod=StandardAxis  RotationAngleUnits=deg  RotationStandardAxis=+X  RotationAngle=90  RotationArbitraryAxis=[0 0 1]  FollAlignAxisA=+X  BaseAlignAxisA=+Y  FollAlignAxisB=+Y  BaseAlignAxisB=+Z  RotationSequenceAxes=FollowerAxes  RotationSequence=XYX  RotationSequenceAngles=[0 0 0]  RotationSequenceAnglesUnits=deg  RotationMatrix=[1 0 0; 0 1 0; 0 0 1]  BlockFunction=simmechanics.library.frames_transforms.rigid_transform
  Conn1 : PMIOPort  Port=1  Side=Right
  connections:
  Rigid Transform8/RConn1 -- Rail2/RConn1
  Rigid Transform11/LConn1 -- Rigid Transform12/RConn1
  Rigid Transform8/LConn1 -- Rigid Transform11/RConn1
  Rigid Transform12/LConn1 -- Conn1/RConn1

== system SimscapeCrane_MPChard/Crane1/XY actuator/X rail/RAIL /Aesthetics/Motor ==
  MotorGearbox : sm_lib/Body Elements/Solid  InertiaType=PointMass  Mass=0  MassUnits=kg  CenterOfMass=[0 0 0]  CenterOfMassUnits=m  MomentsOfInertia=[1 1 1]  MomentsOfInertiaUnits=kg*m^2  ProductsOfInertia=[0 0 0]  ProductsOfInertiaUnits=kg*m^2  DensityBased=off  Density=1000  DensityUnits=kg/(m^3)  DoExposeReferenceFrame=on  SerializedFrames=<Frames/>  GraphicType=FromGeometry  MarkerShape=Sphere  MarkerSize=10  MarkerSizeUnits=m  GraphicVisPropType=SimpleVisualProperties  GraphicDiffuseColor=[0.4 0.4 0.4]  GraphicSpecularColor=[0.5 0.5 0.5 1.0]  GraphicAmbientColor=[0.15 0.15 0.15 1.0]  GraphicEmissiveColor=[0.0 0.0 0.0 1.0]  GraphicShininess=75  GraphicOpacity=1.0  GeometryShape=Cylinder  RectangleSize=[1 1]  RectangleSizeUnits=m  BrickDimensions=[0.06 0.12 0.12]  BrickDimensionUnits=m  CylinderRadius=2.6  CylinderRadiusUnits=cm  CylinderLength=3  CylinderLengthUnits=cm  SphereRadius=1  SphereRadiusUnits=m  EllipsoidRadii=[1 1 1]  EllipsoidRadiiUnits=m  ExtrusionCrossSection=[1 1; -1 1; -1 -1; 1 -1]  ExtrusionCrossSectionUnits=m  ExtrusionLength=1  ExtrusionLengthUnits=m  PolygonNumSides=3  PolygonOuterRadius=1  PolygonOuterRadiusUnits=m  ExtGeomFileType=STL  ExtGeomFileUnits=m  RevolutionCrossSection=[1 1; 1 -1; 2 -1; 2 1]  RevolutionCrossSectionUnits=m  RevolutionExtent=Full  RevolutionAngle=180  RevolutionAngleUnits=deg  BlockFunction=simmechanics.library.body_elements.solid
  Rigid Transform3 : sm_lib/Frames and Transforms/Rigid Transform  TranslationMethod=None  TranslationLengthUnit=m  TranslationStandardAxis=-X  TranslationStandardOffset=0.04  TranslationCartesianOffset="[-0.5 0  0]"  TranslationROffset=0  TranslationROffsetUnits=m  TranslationZOffset=0  TranslationZOffsetUnits=m  TranslationThetaOffset=0  TranslationThetaOffsetUnits=deg  RotationMethod=StandardAxis  RotationAngleUnits=deg  RotationStandardAxis=-X  RotationAngle=90  RotationArbitraryAxis=[0 0 1]  FollAlignAxisA=+X  BaseAlignAxisA=+Y  FollAlignAxisB=+Y  BaseAlignAxisB=+Z  RotationSequenceAxes=FollowerAxes  RotationSequence=XYX  RotationSequenceAngles=[0 0 0]  RotationSequenceAnglesUnits=deg  RotationMatrix=[1 0 0; 0 1 0; 0 0 1]  BlockFunction=simmechanics.library.frames_transforms.rigid_transform
  Rigid Transform4 : sm_lib/Frames and Transforms/Rigid Transform  TranslationMethod=None  TranslationLengthUnit=m  TranslationStandardAxis=-X  TranslationStandardOffset=0.04  TranslationCartesianOffset="[-0.5 0  0]"  TranslationROffset=0  TranslationROffsetUnits=m  TranslationZOffset=0  TranslationZOffsetUnits=m  TranslationThetaOffset=0  TranslationThetaOffsetUnits=deg  RotationMethod=StandardAxis  RotationAngleUnits=deg  RotationStandardAxis=-X  RotationAngle=90  RotationArbitraryAxis=[0 0 1]  FollAlignAxisA=+X  BaseAlignAxisA=+Y  FollAlignAxisB=+Y  BaseAlignAxisB=+Z  RotationSequenceAxes=FollowerAxes  RotationSequence=XYX  RotationSequenceAngles=[0 0 0]  RotationSequenceAnglesUnits=deg  RotationMatrix=[1 0 0; 0 1 0; 0 0 1]  BlockFunction=simmechanics.library.frames_transforms.rigid_transform
  Rigid Transform5 : sm_lib/Frames and Transforms/Rigid Transform  TranslationMethod=StandardAxis  TranslationLengthUnit=m  TranslationStandardAxis=-Y  TranslationStandardOffset=0.015  TranslationCartesianOffset="[-0.5 0  0]"  TranslationROffset=0  TranslationROffsetUnits=m  TranslationZOffset=0  TranslationZOffsetUnits=m  TranslationThetaOffset=0  TranslationThetaOffsetUnits=deg  RotationMethod=None  RotationAngleUnits=deg  RotationStandardAxis=-X  RotationAngle=90  RotationArbitraryAxis=[0 0 1]  FollAlignAxisA=+X  BaseAlignAxisA=+Y  FollAlignAxisB=+Y  BaseAlignAxisB=+Z  RotationSequenceAxes=FollowerAxes  RotationSequence=XYX  RotationSequenceAngles=[0 0 0]  RotationSequenceAnglesUnits=deg  RotationMatrix=[1 0 0; 0 1 0; 0 0 1]  BlockFunction=simmechanics.library.frames_transforms.rigid_transform
  Rigid Transform6 : sm_lib/Frames and Transforms/Rigid Transform  TranslationMethod=StandardAxis  TranslationLengthUnit=m  TranslationStandardAxis=+Y  TranslationStandardOffset=0.03  TranslationCartesianOffset="[-0.5 0  0]"  TranslationROffset=0  TranslationROffsetUnits=m  TranslationZOffset=0  TranslationZOffsetUnits=m  TranslationThetaOffset=0  TranslationThetaOffsetUnits=deg  RotationMethod=None  RotationAngleUnits=deg  RotationStandardAxis=-X  RotationAngle=90  RotationArbitraryAxis=[0 0 1]  FollAlignAxisA=+X  BaseAlignAxisA=+Y  FollAlignAxisB=+Y  BaseAlignAxisB=+Z  RotationSequenceAxes=FollowerAxes  RotationSequence=XYX  RotationSequenceAngles=[0 0 0]  RotationSequenceAnglesUnits=deg  RotationMatrix=[1 0 0; 0 1 0; 0 0 1]  BlockFunction=simmechanics.library.frames_transforms.rigid_transform
  motorBlack : sm_lib/Body Elements/Solid  InertiaType=PointMass  Mass=0  MassUnits=kg  CenterOfMass=[0 0 0]  CenterOfMassUnits=m  MomentsOfInertia=[1 1 1]  MomentsOfInertiaUnits=kg*m^2  ProductsOfInertia=[0 0 0]  ProductsOfInertiaUnits=kg*m^2  DensityBased=off  Density=1000  DensityUnits=kg/(m^3)  DoExposeReferenceFrame=on  SerializedFrames=<Frames/>  GraphicType=FromGeometry  MarkerShape=Sphere  MarkerSize=10  MarkerSizeUnits=m  GraphicVisPropType=AdvancedVisualProperties  GraphicDiffuseColor=[0.1 0.1 0.0]  GraphicSpecularColor=[0.5 0.5 0.5 1.0]  GraphicAmbientColor=[0.15 0.2 0.3 1.0]  GraphicEmissiveColor=[0.0 0.0 0.0 1.0]  GraphicShininess=30  GraphicOpacity=1.0  GeometryShape=Cylinder  RectangleSize=[1 1]  RectangleSizeUnits=m  BrickDimensions=[0.06 0.12 0.12]  BrickDimensionUnits=m  CylinderRadius=1.7  CylinderRadiusUnits=cm  CylinderLength=6  CylinderLengthUnits=cm  SphereRadius=1  SphereRadiusUnits=m  EllipsoidRadii=[1 1 1]  EllipsoidRadiiUnits=m  ExtrusionCrossSection=[1 1; -1 1; -1 -1; 1 -1]  ExtrusionCrossSectionUnits=m  ExtrusionLength=1  ExtrusionLengthUnits=m  PolygonNumSides=3  PolygonOuterRadius=1  PolygonOuterRadiusUnits=m  ExtGeomFileType=STL  ExtGeomFileUnits=m  RevolutionCrossSection=[1 1; 1 -1; 2 -1; 2 1]  RevolutionCrossSectionUnits=m  RevolutionExtent=Full  RevolutionAngle=180  RevolutionAngleUnits=deg  BlockFunction=simmechanics.library.body_elements.solid
  Conn1 : PMIOPort  Port=1  Side=Left
  connections:
  Rigid Transform3/RConn1 -- motorBlack/RConn1
  Rigid Transform4/RConn1 -- MotorGearbox/RConn1
  Rigid Transform5/LConn1 -- Rigid Transform6/LConn1 -- Conn1/RConn1
  Rigid Transform6/RConn1 -- Rigid Transform4/LConn1
  Rigid Transform5/RConn1 -- Rigid Transform3/LConn1

== matlab function SimscapeCrane_MPChard/MPC/MPC ==
  data: Al input; blx0 input; u output; Qbar input; ucon input; x0 input; xTarget input; m input; N input; Dx0 input; CD input
function u  = myLPController(Al,blx0,Qbar,ucon,x0,xTarget,m,N,Dx0,CD)
% H       - quadratic term in the cost function.
% G       - matrix in the linear term in the cost function.
% F       - LHS of the inequalities term.
% bb      - RHS of the inequalities term.
% J       - RHS of inequalities term.
% L       - RHS of inequalities term. Use this to shift constraints around target point
% x       - current state
% xTarget - target equilibrium point.
% m       - Number of inputs.
% iA      - active inequalities, see doc mpcqpsolver
%
% u is the first input vector u_0 in the sequence [u_0; u_1; ...; u_{N-1}]; 
% In other words, u is the value of the receding horizon control law
% evaluated with the current state x0 and target xTarget
%% your code starts here
options = optimoptions('linprog','Algorithm','dual-simplex');
options.MaxIter=1000;
ft=[zeros(1,m*N) ones(1,N*8+m*N)];
%b=[blx0*x0+blxe*xTarget;ucon;Dx0*x0+CD];
blxe=[-Qbar*kron(ones(N,1),xTarget);zeros(N*m,1);Qbar*kron(ones(N,1),xTarget);zeros(N*m,1)];
b=[blx0*x0-blxe;ucon];

[U,~,~]=linprog(ft,Al,b,[],[],[],[],x0,options);
%% your remaining code here
u=U(1:m);
end
